simulink library "rwa_allocation_lib"  (R2018b)
settings: Solver=VariableStepAuto  StartTime=0.0  StopTime=10.0  RelTol=1e-3
undefined symbols (not defined in the file): DiscIntNeverNeededParam, fswParams
libraries: L_inf_allocation_lib x2, aerolibutil x1
settings Model: Creator=taylorreynolds  LastModifiedBy=Taylor

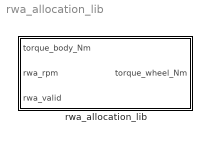
== system rwa_allocation_lib ==
  rwa_allocation_lib : Subsystem  TreatAsAtomicUnit=on
      settings: RTWFcnNameOpts=Use subsystem name  RTWFileNameOpts=Use subsystem name

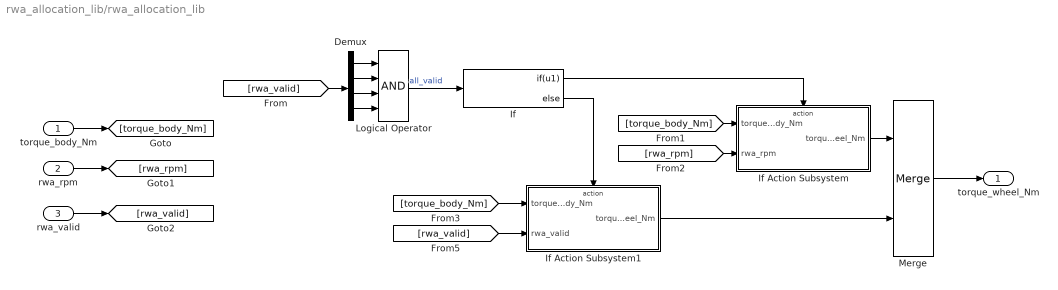
== system rwa_allocation_lib/rwa_allocation_lib ==
  torque_body_Nm : Inport
  rwa_rpm : Inport  Port=2
  rwa_valid : Inport  Port=3
  Demux : Demux
  If : If  IfExpression=u1
  If Action Subsystem : Subsystem  TreatAsAtomicUnit=on
  If Action Subsystem1 : Subsystem  TreatAsAtomicUnit=on
  Logical Operator : Logic  Inputs=4  AllPortsSameDT=off  OutDataTypeStr=boolean
  Merge : Merge
  torque_wheel_Nm : Outport
  wires:
  Demux/1 -> Logical Operator/1
  Demux/2 -> Logical Operator/2
  Demux/3 -> Logical Operator/3
  Demux/4 -> Logical Operator/4
  Logical Operator/1 -> If/1  "all_valid"
  If Action Subsystem/1(torque_wheel_Nm) -> Merge/1
  If Action Subsystem1/1(torque_wheel_Nm) -> Merge/2
  Merge/1 -> torque_wheel_Nm/1
  torque_body_Nm/1 -> [torque_body_Nm]
  rwa_rpm/1 -> [rwa_rpm]
  rwa_valid/1 -> [rwa_valid]
  [rwa_valid] -> Demux/1
  If/1 -> If Action Subsystem/Action
  If/2 -> If Action Subsystem1/Action
  [torque_body_Nm] -> If Action Subsystem/1(torque_body_Nm)
  [rwa_rpm] -> If Action Subsystem/2(rwa_rpm)
  [torque_body_Nm] -> If Action Subsystem1/1(torque_body_Nm)
  [rwa_valid] -> If Action Subsystem1/2("rwa_valid ")

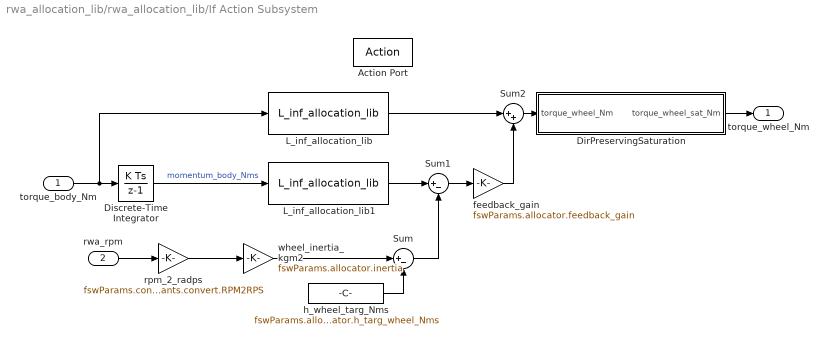
== system rwa_allocation_lib/rwa_allocation_lib/If Action Subsystem ==
  torque_body_Nm : Inport
  rwa_rpm : Inport  Port=2
  Action Port : ActionPort  ActionType=then
  DirPreservingSaturation : Subsystem
  Discrete-Time Integrator : DiscreteIntegrator  SampleTime=-1  ICPrevOutput=DiscIntNeverNeededParam  ICPrevScaledInput=DiscIntNeverNeededParam
  L_inf_allocation_lib : L_inf_allocation_lib/L_inf_allocation_lib  SystemSampleTime=-1
  L_inf_allocation_lib1 : L_inf_allocation_lib/L_inf_allocation_lib  SystemSampleTime=-1
  Sum : Sum  Inputs=|+-
  Sum1 : Sum  Inputs=|+-
  Sum2 : Sum  Inputs=|++
  feedback_gain : Gain  Gain=fswParams.allocator.feedback_gain
  h_wheel_targ_Nms : Constant  Value=fswParams.allocator.h_targ_wheel_Nms
  rpm_2_radps : Gain  Gain=fswParams.constants.convert.RPM2RPS
  wheel_inertia_kgm2 : Gain  Gain=fswParams.allocator.inertia
  torque_wheel_Nm : Outport
  wires:
  h_wheel_targ_Nms/1 -> Sum/2
  wheel_inertia_kgm2/1 -> Sum/1
  rpm_2_radps/1 -> wheel_inertia_kgm2/1
  Discrete-Time Integrator/1 -> L_inf_allocation_lib1/1  "momentum_body_Nms"
  L_inf_allocation_lib1/1 -> Sum1/1
  L_inf_allocation_lib/1 -> Sum2/1
  torque_body_Nm/1 -> Discrete-Time Integrator/1, L_inf_allocation_lib/1
  rwa_rpm/1 -> rpm_2_radps/1
  Sum2/1 -> DirPreservingSaturation/1(torque_wheel_Nm)
  Sum1/1 -> feedback_gain/1
  Sum/1 -> Sum1/2
  feedback_gain/1 -> Sum2/2
  DirPreservingSaturation/1(torque_wheel_sat_Nm) -> torque_wheel_Nm/1

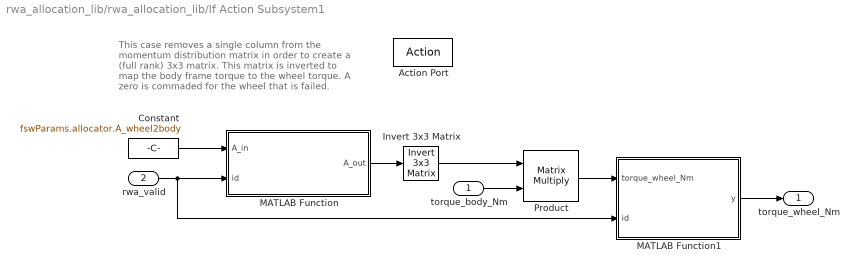
== system rwa_allocation_lib/rwa_allocation_lib/If Action Subsystem1 ==
  note: This case removes a single column from the
      | momentum distribution matrix in order to create
      | a (full rank) 3x3 matrix. This matrix is inverted to
      | map the body frame torque to the wheel torque.
      | A zero is commaded for the wheel that is failed.
  torque_body_Nm : Inport
  "rwa_valid " : Inport  Port=2
  Action Port : ActionPort  ActionType=else
  Constant : Constant  Value=fswParams.allocator.A_wheel2body
  Invert 3x3 Matrix : aerolibutil/Invert  3x3 Matrix
  MATLAB Function : MATLAB Function  TreatAsAtomicUnit=on
  MATLAB Function1 : MATLAB Function  TreatAsAtomicUnit=on
  Product : Product  Multiplication=Matrix(*)
  torque_wheel_Nm : Outport
  wires:
  Constant/1 -> MATLAB Function/1(A_in)
  MATLAB Function/1(A_out) -> Invert 3x3 Matrix/1
  Invert 3x3 Matrix/1 -> Product/1
  torque_body_Nm/1 -> Product/2
  Product/1 -> MATLAB Function1/1(torque_wheel_Nm)
  "rwa_valid "/1 -> MATLAB Function/2(id), MATLAB Function1/2(id)
  MATLAB Function1/1(y) -> torque_wheel_Nm/1

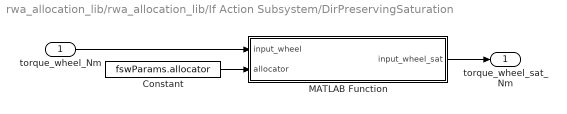
== system rwa_allocation_lib/rwa_allocation_lib/If Action Subsystem/DirPreservingSaturation ==
  torque_wheel_Nm : Inport
  Constant : Constant  Value=fswParams.allocator  OutDataTypeStr=Bus: RWA
  MATLAB Function : MATLAB Function  TreatAsAtomicUnit=on
  torque_wheel_sat_Nm : Outport
  wires:
  MATLAB Function/1(input_wheel_sat) -> torque_wheel_sat_Nm/1
  torque_wheel_Nm/1 -> MATLAB Function/1(input_wheel)
  Constant/1 -> MATLAB Function/2(allocator)

== matlab function rwa_allocation_lib/If Action Subsystem1/MATLAB Function1 ==
  data: torque_wheel_Nm input size=3; y output size=4; id input size=4
function y = assign_torque(torque_wheel_Nm,id)

y = zeros(4,1);

n_whl = uint8(0);
for k = 1:4
   if (id(k))
       n_whl = n_whl + 1;
       y(k) = torque_wheel_Nm(n_whl);
   end
end

end

== matlab function rwa_allocation_lib/If Action Subsystem1/MATLAB Function ==
  data: A_in input double size=3,4; A_out output size=3,3; id input boolean size=4
function A_out = get_alloc_matrix(A_in,id)
%#codegen

num_good = uint8(sum(id));

switch num_good
    
    case {0,1,2}
        % just output the identity
        A_out = eye(3);
        
    case 3
        % extract the columns of the allocation matrix for the un-failed
        % wheels (the "good" wheels)
        id_good = zeros(3,1);   
        n_whl = 1;
        for k = 1:4
            if (id(k))
                id_good(n_whl) = k;
                n_whl = n_whl + 1;
            end
        end
        A_out = A_in(:,id_good);
        
    case 4
        % just take the first three columns, no sweat since the other
        % allocation scheme will be chosen anyway. This is just to handle
        % an annoying simulink thing in that it checks every possible
        % thread of execution before running & can't distinguish that this
        % case will never get used
        A_out = A_in(:,1:3);
        
    otherwise
        A_out = eye(3);
end

end

== matlab function rwa_allocation_lib/If Action Subsystem/DirPreservingSaturation/MATLAB Function ==
  data: input_wheel input; input_wheel_sat output; allocator input Bus: RWA
function input_wheel_sat = fcn(input_wheel,allocator)
%#codegen

In = eye(4);
A = [ In; -In ];

temp = A*input_wheel-allocator.max_torque_Nm;
[val,id] = max(temp);

a = A(id,:);
b = allocator.max_torque_Nm;
c = dot(a,input_wheel);

if ( val > 0 )
    input_wheel_sat = (b/c) .* input_wheel;
else
    input_wheel_sat = input_wheel;
end

end
